simulink model "ekf2sim"  (R2014a)
settings: Solver=FixedStepDiscrete  StartTime=0.0  StopTime=100.0  RelTol=1e-3
values from neighbouring files (symbols this model uses):
  T = block.DialogPrm(6).Data    [sfall2.m]    (also in sysall.m = 0.05)
undefined symbols (not defined in the file): phi_0, psi_0, Q, R, theta_0, V_0
libraries: simulink x3
CloseFcn:
  | rtwprivate ssgensfun ModelCloseRequest ekfv63
settings Model: Creator=stefy  LastModifiedBy=gcampa
settings DataIOCC: SignalLoggingSaveFormat=ModelDataLogs  SaveOutput=off  SignalLogging=off  DSMLogging=off  SaveTime=off
settings OptimizationCC: ExpressionDepthLimit=2147483647  InitFltsAndDblsToZero=on
settings DebuggingCC: SaveWithParameterizedLinksMsg=none  UnderspecifiedInitializationDetection=Classic  SignalResolutionControl=TryResolveAllWithWarning  MultiTaskDSMMsg=warning  MultiTaskCondExecSysMsg=none  FcnCallInpInsideContextMsg=UseLocalSettings  StateNameClashWarn=warning
settings SFSimCC: SimParseCustomCode=off
settings RTWCC: IncludeERTFirstTime=on  RTWCompilerOptimization=On
settings GRTTargetCC: TargetFcnLib=ansi_tfl_tmw.mat  CombineOutputUpdateFcns=off  GRTInterface=on

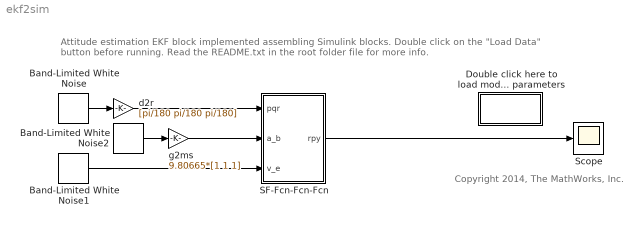
== system ekf2sim ==
  note: Attitude estimation EKF block implemented assembling Simulink blocks.
      | Double click on the "Load Data" button before running. Read the README.txt in the root folder file for more info.
  note: Copyright 2014, The MathWorks, Inc.
  Band-Limited White Noise : simulink/Sources/Band-Limited White Noise  Cov=0.1*[1 1 1]  Ts=T  seed=[1 2 3]
  Band-Limited White Noise1 : simulink/Sources/Band-Limited White Noise  Cov=0.1*[1 1 1]  Ts=T  seed=[7 8 9]
  Band-Limited White Noise2 : simulink/Sources/Band-Limited White Noise  Cov=0.1*[1 1 1]  Ts=T  seed=[4 5 6]
  Double click here to load model and parameters : Subsystem
      settings: OpenFcn=|
      | V_0= 21.44176640107837;
      | phi_0=0.16673723163960;
      | theta_0=0.38249284705297;
      | psi_0=-3.10672050096899;
      | 
      | Q= [1.1339e-006     0               0
      |     0               3.1232e-006     0
      |     0               0               2.9009e-006];
      | 
      | R= [0.3368          0               0
      |     0               0.092           0
      |     0               0               0];
      | 
      | T=0.05;
      mask Display: disp('Load\nData')
  SF-Fcn-Fcn-Fcn : Subsystem
  Scope : Scope
      settings: TimeRange=100  YMin=-4  YMax=4
  d2r : Gain  Gain=[pi/180 pi/180 pi/180]  SaturateOnIntegerOverflow=on  OutDataTypeStr=Inherit: Same as input  ParamDataTypeStr=Inherit: Same as input
  g2ms : Gain  Gain=9.80665*[1 1 1]  SaturateOnIntegerOverflow=on  OutDataTypeStr=Inherit: Same as input  ParamDataTypeStr=Inherit: Same as input
  wires:
  Band-Limited White Noise/1 -> d2r/1
  Band-Limited White Noise1/1 -> SF-Fcn-Fcn-Fcn/3(v_e)
  Band-Limited White Noise2/1 -> g2ms/1
  SF-Fcn-Fcn-Fcn/1(rpy) -> Scope/1
  d2r/1 -> SF-Fcn-Fcn-Fcn/1(pqr)
  g2ms/1 -> SF-Fcn-Fcn-Fcn/2(a_b)

== system ekf2sim/Double click here to load model and parameters ==

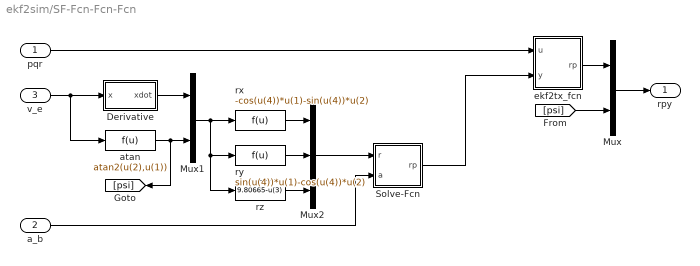
== system ekf2sim/SF-Fcn-Fcn-Fcn ==
  pqr : Inport
  a_b : Inport  Port=2
  v_e : Inport  Port=3
  Derivative : Subsystem  mask(Time Derivative){T=T, x0=[V_0*cos(psi_0) V_0*sin(psi_0) V_0*sin(theta_0)]}
      mask prompts: T "Sampling Time"; x0 "Initial Condition"
      mask help:
      | First order approximation of the time derivative of the input signal,
      |   the original one is buggy.
  Mux : Mux  Inputs=[2 1]
  Mux1 : Mux  Inputs=[3 1]
  Mux2 : Mux  Inputs=[1 1 1]
  Solve-Fcn : Subsystem
  atan : Fcn  Expr=atan2(u(2),u(1))  SampleTime=T
  ekf2tx_fcn : Subsystem  mask(Extended Kalman Filter){W=Q(1:2,1:2), V=R(1:2,1:2), x0=[phi_0 theta_0]', P0=zeros(2), Plim=1e-5, T=T}
      mask prompts: Plim "P limiter"; T "Sample Time"
      mask help: Milimalistic 2-states Extended Kalman Filter for attitude estimation
  rx : Fcn  Expr=-cos(u(4))*u(1)-sin(u(4))*u(2)
  ry : Fcn  Expr=sin(u(4))*u(1)-cos(u(4))*u(2)
  rz : Fcn  Expr=9.80665-u(3)
  rpy : Outport
  wires:
  v_e/1 -> atan/1, Derivative/1(x)
  rz/1 -> Mux2/3
  Mux2/1 -> Solve-Fcn/1(r)
  ry/1 -> Mux2/2
  rx/1 -> Mux2/1
  atan/1 -> [psi], Mux1/2
  Derivative/1(xdot) -> Mux1/1
  Mux1/1 -> rz/1, ry/1, rx/1
  [psi] -> Mux/2
  ekf2tx_fcn/1(rp) -> Mux/1
  Solve-Fcn/1(rp) -> ekf2tx_fcn/2(y)
  a_b/1 -> Solve-Fcn/2(a)
  pqr/1 -> ekf2tx_fcn/1(u)
  Mux/1 -> rpy/1

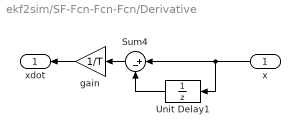
== system ekf2sim/SF-Fcn-Fcn-Fcn/Derivative ==
  x : Inport  SampleTime=T
  Sum4 : Sum  Inputs=|+-  SaturateOnIntegerOverflow=on  InputSameDT=on  OutDataTypeStr=Inherit: Same as first input
  Unit Delay1 : UnitDelay  InitialCondition=x0  SampleTime=T
  gain : Gain  Gain=1/T  SampleTime=T  SaturateOnIntegerOverflow=on  OutDataTypeStr=Inherit: Same as input  ParamDataTypeStr=Inherit: Same as input
  xdot : Outport
  wires:
  gain/1 -> xdot/1
  x/1 -> Unit Delay1/1, Sum4/1
  Unit Delay1/1 -> Sum4/2
  Sum4/1 -> gain/1

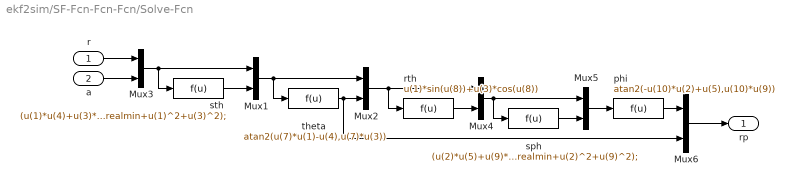
== system ekf2sim/SF-Fcn-Fcn-Fcn/Solve-Fcn ==
  r : Inport
  a : Inport  Port=2
  Mux1 : Mux  Inputs=[6 1]
  Mux2 : Mux  Inputs=[7 1]
  Mux3 : Mux  Inputs=[3 3]
  Mux4 : Mux  Inputs=[8 1]
  Mux5 : Mux  Inputs=[9 1]
  Mux6 : Mux  Inputs=[1 1]
  phi : Fcn  Expr=atan2(-u(10)*u(2)+u(5),u(10)*u(9))
  rth : Fcn  Expr=u(1)*sin(u(8))+u(3)*cos(u(8))
  sph : Fcn  Expr=(u(2)*u(5)+u(9)*(abs(u(2)^2+u(9)^2-u(5)^2)^0.5))/(realmin+u(2)^2+u(9)^2);
  sth : Fcn  Expr=(u(1)*u(4)+u(3)*(abs(u(1)^2+u(3)^2-u(4)^2)^0.5))/(realmin+u(1)^2+u(3)^2);
  theta : Fcn  Expr=atan2(u(7)*u(1)-u(4),u(7)*u(3))
  rp : Outport
  wires:
  Mux6/1 -> rp/1
  phi/1 -> Mux6/1
  Mux5/1 -> phi/1
  sph/1 -> Mux5/2
  Mux4/1 -> Mux5/1, sph/1
  rth/1 -> Mux4/2
  Mux2/1 -> Mux4/1, rth/1
  theta/1 -> Mux6/2, Mux2/2
  Mux1/1 -> Mux2/1, theta/1
  sth/1 -> Mux1/2
  a/1 -> Mux3/2
  r/1 -> Mux3/1
  Mux3/1 -> Mux1/1, sth/1

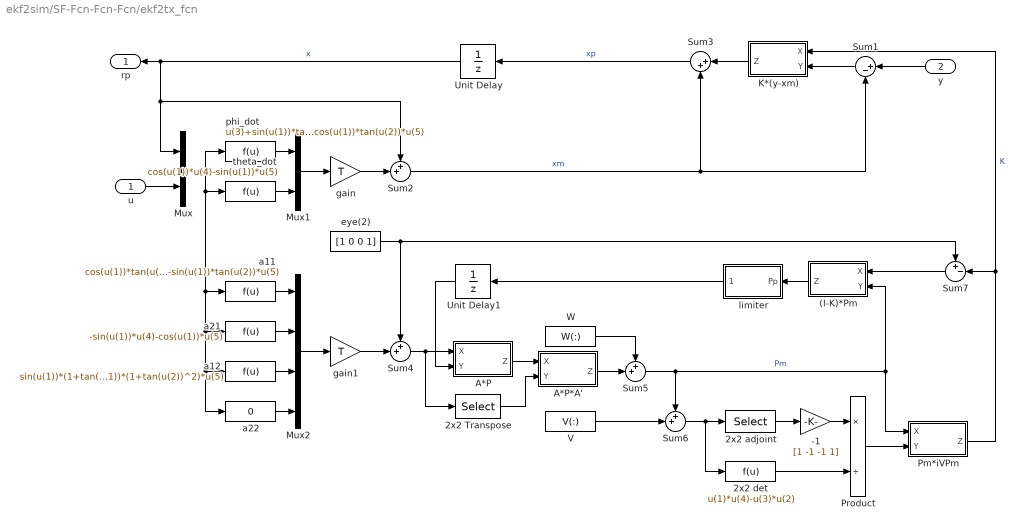
== system ekf2sim/SF-Fcn-Fcn-Fcn/ekf2tx_fcn ==
  u : Inport
  y : Inport  Port=2
  (I-K)*Pm : Subsystem  mask(2x2 Matrix Multiplication){}
      mask help:
      | Input 1   : elements of matrix X (2 by 2)
      |   Input 2   : elements of matrix Y (2 by 2)
      |   Output   : elements of matrix X*Y (2 by 2)
      mask Help:
      | <p>
      | Elements of input and output matrices are taken columnwise.
      | </p>
      mask Display: disp('Z=X*Y')
  -1 : Gain  Gain=[1 -1 -1 1]  SaturateOnIntegerOverflow=on  OutDataTypeStr=Inherit: Same as input  ParamDataTypeStr=Inherit: Same as input
  2x2 Transpose : Selector  InputPortWidth=4  Indices=[1 3 2 4]
  2x2 adjoint : Selector  InputPortWidth=4  Indices=[4 2 3 1]
  2x2 det : Fcn  Expr=u(1)*u(4)-u(3)*u(2)
  A*P : Subsystem  mask(2x2 Matrix Multiplication){}
      mask help:
      | Input 1   : elements of matrix X (2 by 2)
      |   Input 2   : elements of matrix Y (2 by 2)
      |   Output   : elements of matrix X*Y (2 by 2)
      mask Help:
      | <p>
      | Elements of input and output matrices are taken columnwise.
      | </p>
      mask Display: disp('Z=X*Y')
  A*P*A' : Subsystem  mask(2x2 Matrix Multiplication){}
      mask help:
      | Input 1   : elements of matrix X (2 by 2)
      |   Input 2   : elements of matrix Y (2 by 2)
      |   Output   : elements of matrix X*Y (2 by 2)
      mask Help:
      | <p>
      | Elements of input and output matrices are taken columnwise.
      | </p>
      mask Display: disp('Z=X*Y')
  K*(y-xm) : Subsystem  mask(2x2 Matrix Multiplication){}
      mask help:
      | Input 1   : elements of matrix X (2 by 2)
      |   Input 2   : elements of matrix Y (2 by 2)
      |   Output   : elements of matrix X*Y (2 by 2)
      mask Help:
      | <p>
      | Elements of input and output matrices are taken columnwise.
      | </p>
      mask Display: disp('Z=X*Y')
  Mux : Mux  Inputs=[2 3]
  Mux1 : Mux  Inputs=[1 1]
  Mux2 : Mux  Inputs=[1 1 1 1]
  Pm*iVPm : Subsystem  mask(2x2 Matrix Multiplication){}
      mask help:
      | Input 1   : elements of matrix X (2 by 2)
      |   Input 2   : elements of matrix Y (2 by 2)
      |   Output   : elements of matrix X*Y (2 by 2)
      mask Help:
      | <p>
      | Elements of input and output matrices are taken columnwise.
      | </p>
      mask Display: disp('Z=X*Y')
  Product : Product  Inputs=*/  RndMeth=Zero
  Sum1 : Sum  Inputs=|+-  SaturateOnIntegerOverflow=on  InputSameDT=on  OutDataTypeStr=Inherit: Same as first input
  Sum{2,4..6} (4 alike) : Sum  Inputs=++|  SaturateOnIntegerOverflow=on  InputSameDT=on  OutDataTypeStr=Inherit: Same as first input
  Sum3 : Sum  Inputs=|++  SaturateOnIntegerOverflow=on  InputSameDT=on  OutDataTypeStr=Inherit: Same as first input
  Sum7 : Sum  Inputs=+-|  SaturateOnIntegerOverflow=on  InputSameDT=on  OutDataTypeStr=Inherit: Same as first input
  Unit Delay : UnitDelay  InitialCondition=x0  SampleTime=T
  Unit Delay1 : UnitDelay  InitialCondition=P0(:)  SampleTime=T
  V : Constant  Value=V(:)
  W : Constant  Value=W(:)
  a11 : Fcn  Expr=cos(u(1))*tan(u(2))*u(4)-sin(u(1))*tan(u(2))*u(5)
  a12 : Fcn  Expr=sin(u(1))*(1+tan(u(2))^2)*u(4)+cos(u(1))*(1+tan(u(2))^2)*u(5)
  a21 : Fcn  Expr=-sin(u(1))*u(4)-cos(u(1))*u(5)
  a22 : Fcn  Expr=0
  eye(2) : Constant  Value=[1 0 0 1]
  gain : Gain  Gain=T  SaturateOnIntegerOverflow=on  OutDataTypeStr=Inherit: Same as input  ParamDataTypeStr=Inherit: Same as input
  gain1 : Gain  Gain=T  SampleTime=T  SaturateOnIntegerOverflow=on  OutDataTypeStr=Inherit: Same as input  ParamDataTypeStr=Inherit: Same as input
  limiter : Subsystem
  phi_dot : Fcn  Expr=u(3)+sin(u(1))*tan(u(2))*u(4)+cos(u(1))*tan(u(2))*u(5)
  theta_dot : Fcn  Expr=cos(u(1))*u(4)-sin(u(1))*u(5)
  rp : Outport
  wires:
  Sum2/1 -> Sum3/2, Sum1/2  "xm"
  gain/1 -> Sum2/2
  Mux1/1 -> gain/1
  phi_dot/1 -> Mux1/1
  theta_dot/1 -> Mux1/2
  Mux/1 -> phi_dot/1, theta_dot/1, a22/1, a12/1, a21/1, a11/1
  Unit Delay/1 -> Mux/1, Sum2/1, rp/1  "x"
  u/1 -> Mux/2
  y/1 -> Sum1/1
  Sum3/1 -> Unit Delay/1  "xp"
  a11/1 -> Mux2/1
  a21/1 -> Mux2/2
  a12/1 -> Mux2/3
  a22/1 -> Mux2/4
  Mux2/1 -> gain1/1
  gain1/1 -> Sum4/2
  eye(2)/1 -> Sum4/1, Sum7/1
  Sum4/1 -> A*P/1(X), 2x2 Transpose/1
  A*P/1(Z) -> A*P*A'/1(X)
  2x2 Transpose/1 -> A*P*A'/2(Y)
  Unit Delay1/1 -> A*P/2(Y)
  A*P*A'/1(Z) -> Sum5/2
  W/1 -> Sum5/1
  Sum5/1 -> Sum6/1, Pm*iVPm/1(X), (I-K)*Pm/2(Y)  "Pm"
  Sum6/1 -> 2x2 det/1, 2x2 adjoint/1
  2x2 adjoint/1 -> -1/1
  2x2 det/1 -> Product/2
  -1/1 -> Product/1
  Product/1 -> Pm*iVPm/2(Y)
  V/1 -> Sum6/2
  Pm*iVPm/1(Z) -> Sum7/2, K*(y-xm)/1(X)  "K"
  Sum7/1 -> (I-K)*Pm/1(X)
  K*(y-xm)/1(Z) -> Sum3/1
  Sum1/1 -> K*(y-xm)/2(Y)
  limiter/1(ball(Pp)) -> Unit Delay1/1
  (I-K)*Pm/1(Z) -> limiter/1(Pp)

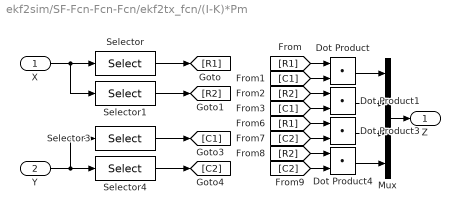
== system ekf2sim/SF-Fcn-Fcn-Fcn/ekf2tx_fcn/(I-K)*Pm ==
  X : Inport
  Y : Inport  Port=2
  Dot Product{,1,3..4} (4 alike) : DotProduct  InputSameDT=on  OutDataTypeStr=Inherit: Inherit via internal rule
  Mux : Mux  Inputs=ones(4,1)
  Selector : Selector  InputPortWidth=4  Indices=[1 3]
  Selector1 : Selector  InputPortWidth=4  Indices=[2 4]
  Selector3 : Selector  InputPortWidth=4  Indices=[1 2]
  Selector4 : Selector  InputPortWidth=4  Indices=[3 4]
  Z : Outport
  wires:
  Mux/1 -> Z/1
  Selector3/1 -> [C1]
  Selector4/1 -> [C2]
  Selector1/1 -> [R2]
  Y/1 -> Selector3/1, Selector4/1
  [C2] -> Dot Product4/2
  [R2] -> Dot Product4/1
  [C2] -> Dot Product3/2
  [R1] -> Dot Product3/1
  [C1] -> Dot Product1/2
  [R2] -> Dot Product1/1
  [C1] -> Dot Product/2
  [R1] -> Dot Product/1
  Selector/1 -> [R1]
  X/1 -> Selector/1, Selector1/1
  Dot Product/1 -> Mux/1
  Dot Product1/1 -> Mux/2
  Dot Product3/1 -> Mux/3
  Dot Product4/1 -> Mux/4

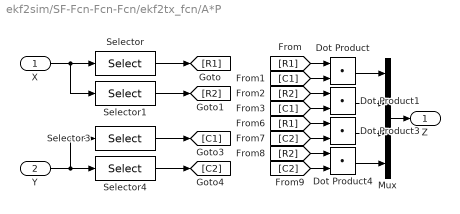
== system ekf2sim/SF-Fcn-Fcn-Fcn/ekf2tx_fcn/A*P ==
  X : Inport
  Y : Inport  Port=2
  Dot Product{,1,3..4} (4 alike) : DotProduct  InputSameDT=on  OutDataTypeStr=Inherit: Inherit via internal rule
  Mux : Mux  Inputs=ones(4,1)
  Selector : Selector  InputPortWidth=4  Indices=[1 3]
  Selector1 : Selector  InputPortWidth=4  Indices=[2 4]
  Selector3 : Selector  InputPortWidth=4  Indices=[1 2]
  Selector4 : Selector  InputPortWidth=4  Indices=[3 4]
  Z : Outport
  wires:
  Mux/1 -> Z/1
  Selector3/1 -> [C1]
  Selector1/1 -> [R2]
  Y/1 -> Selector3/1, Selector4/1
  [C2] -> Dot Product4/2
  [R2] -> Dot Product4/1
  [C2] -> Dot Product3/2
  [R1] -> Dot Product3/1
  [C1] -> Dot Product1/2
  [R2] -> Dot Product1/1
  [C1] -> Dot Product/2
  [R1] -> Dot Product/1
  Selector/1 -> [R1]
  X/1 -> Selector/1, Selector1/1
  Dot Product/1 -> Mux/1
  Dot Product1/1 -> Mux/2
  Dot Product3/1 -> Mux/3
  Dot Product4/1 -> Mux/4
  Selector4/1 -> [C2]

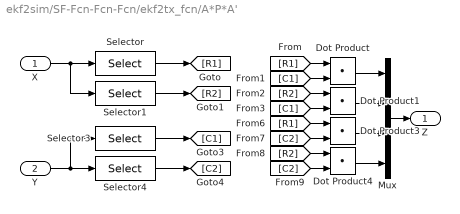
== system ekf2sim/SF-Fcn-Fcn-Fcn/ekf2tx_fcn/A*P*A' ==
  X : Inport
  Y : Inport  Port=2
  Dot Product{,1,3..4} (4 alike) : DotProduct  InputSameDT=on  OutDataTypeStr=Inherit: Inherit via internal rule
  Mux : Mux  Inputs=ones(4,1)
  Selector : Selector  InputPortWidth=4  Indices=[1 3]
  Selector1 : Selector  InputPortWidth=4  Indices=[2 4]
  Selector3 : Selector  InputPortWidth=4  Indices=[1 2]
  Selector4 : Selector  InputPortWidth=4  Indices=[3 4]
  Z : Outport
  wires:
  Dot Product4/1 -> Mux/4
  Dot Product3/1 -> Mux/3
  Dot Product1/1 -> Mux/2
  Dot Product/1 -> Mux/1
  X/1 -> Selector1/1, Selector/1
  Selector/1 -> [R1]
  [R1] -> Dot Product/1
  [C1] -> Dot Product/2
  [R2] -> Dot Product1/1
  [C1] -> Dot Product1/2
  [R1] -> Dot Product3/1
  [C2] -> Dot Product3/2
  [R2] -> Dot Product4/1
  [C2] -> Dot Product4/2
  Y/1 -> Selector4/1, Selector3/1
  Selector1/1 -> [R2]
  Selector4/1 -> [C2]
  Selector3/1 -> [C1]
  Mux/1 -> Z/1

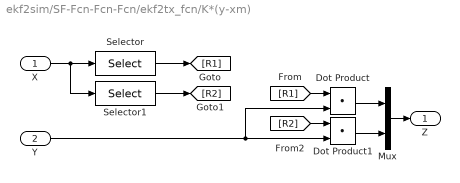
== system ekf2sim/SF-Fcn-Fcn-Fcn/ekf2tx_fcn/K*(y-xm) ==
  X : Inport
  Y : Inport  Port=2
  Dot Product : DotProduct  InputSameDT=on  OutDataTypeStr=Inherit: Inherit via internal rule
  Dot Product1 : DotProduct  InputSameDT=on  OutDataTypeStr=Inherit: Inherit via internal rule
  Mux : Mux  Inputs=ones(2,1)
  Selector : Selector  InputPortWidth=4  Indices=[1 3]
  Selector1 : Selector  InputPortWidth=4  Indices=[2 4]
  Z : Outport
  wires:
  Dot Product1/1 -> Mux/2
  Dot Product/1 -> Mux/1
  X/1 -> Selector1/1, Selector/1
  Selector/1 -> [R1]
  [R1] -> Dot Product/1
  [R2] -> Dot Product1/1
  Y/1 -> Dot Product1/2, Dot Product/2
  Selector1/1 -> [R2]
  Mux/1 -> Z/1

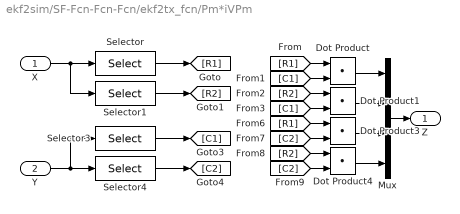
== system ekf2sim/SF-Fcn-Fcn-Fcn/ekf2tx_fcn/Pm*iVPm ==
  X : Inport
  Y : Inport  Port=2
  Dot Product{,1,3..4} (4 alike) : DotProduct  InputSameDT=on  OutDataTypeStr=Inherit: Inherit via internal rule
  Mux : Mux  Inputs=ones(4,1)
  Selector : Selector  InputPortWidth=4  Indices=[1 3]
  Selector1 : Selector  InputPortWidth=4  Indices=[2 4]
  Selector3 : Selector  InputPortWidth=4  Indices=[1 2]
  Selector4 : Selector  InputPortWidth=4  Indices=[3 4]
  Z : Outport
  wires:
  Mux/1 -> Z/1
  Selector3/1 -> [C1]
  Selector4/1 -> [C2]
  Selector1/1 -> [R2]
  Y/1 -> Selector3/1, Selector4/1
  [C2] -> Dot Product4/2
  [R2] -> Dot Product4/1
  [C2] -> Dot Product3/2
  [R1] -> Dot Product3/1
  [C1] -> Dot Product1/2
  [R2] -> Dot Product1/1
  [C1] -> Dot Product/2
  [R1] -> Dot Product/1
  Selector/1 -> [R1]
  X/1 -> Selector/1, Selector1/1
  Dot Product/1 -> Mux/1
  Dot Product1/1 -> Mux/2
  Dot Product3/1 -> Mux/3
  Dot Product4/1 -> Mux/4

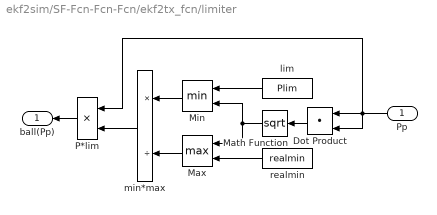
== system ekf2sim/SF-Fcn-Fcn-Fcn/ekf2tx_fcn/limiter ==
  Pp : Inport
  Dot Product : DotProduct  InputSameDT=on  OutDataTypeStr=Inherit: Inherit via internal rule
  Math Function : Math  Operator=sqrt  SaturateOnIntegerOverflow=on
  Max : MinMax  Function=max  Inputs=2
  Min : MinMax  Inputs=2
  P*lim : Product  Inputs=**  RndMeth=Zero
  lim : Constant  Value=Plim
  min*max : Product  Inputs=*/  RndMeth=Zero
  realmin : Constant  Value=realmin
  ball(Pp) : Outport
  wires:
  Pp/1 -> Dot Product/1, Dot Product/2, P*lim/1
  Dot Product/1 -> Math Function/1
  Math Function/1 -> Max/1, Min/2
  P*lim/1 -> ball(Pp)/1
  realmin/1 -> Max/2
  lim/1 -> Min/1
  Min/1 -> min*max/1
  Max/1 -> min*max/2
  min*max/1 -> P*lim/2
